simulink model "heating_system_model"  (R2022b)
settings: Solver=VariableStepAuto  StartTime=0.0  StopTime=500  RelTol=1e-3
model workspace (MAT data in the model file):
  h0 = [0 1 1 0]
  p0 = [0 1 1 0]
  x0 = [16.5 16.5 16.5 16.5]
settings Model: Creator=Cameron  LastModifiedBy=Cameron

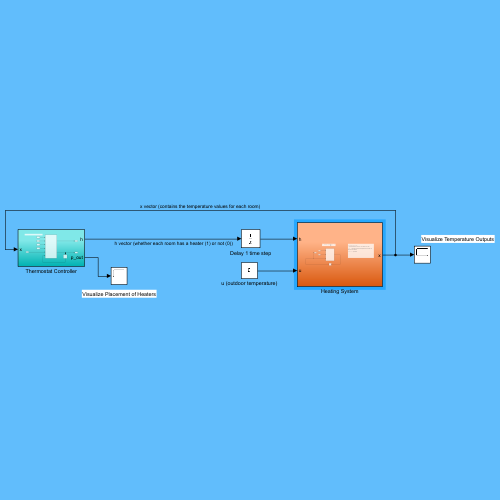
[thumbnail: Simulink's stored preview of the top-level diagram]
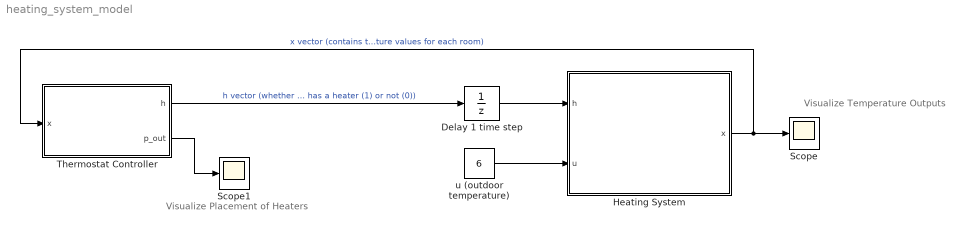
== system heating_system_model ==
  note: Visualize Placement of Heaters
  note: Visualize Temperature Outputs
  Delay 1 time step : UnitDelay  SampleTime=-1  HasFrameUpgradeWarning=on
  Heating System : Subsystem
  Scope : Scope
  Scope1 : Scope
  Thermostat Controller : Subsystem
  u (outdoor temperature) : Constant  Value=6
  wires:
  Thermostat Controller/1(h) -> Delay 1 time step/1  "h vector (whether each room has a heater (1) or not (0))"
  Heating System/1(x) -> Scope/1, Thermostat Controller/1(x)  "x vector (contains the temperature values for each room)"
  u (outdoor temperature)/1 -> Heating System/2(u)
  Delay 1 time step/1 -> Heating System/1(h)
  Thermostat Controller/2(p_out) -> Scope1/1

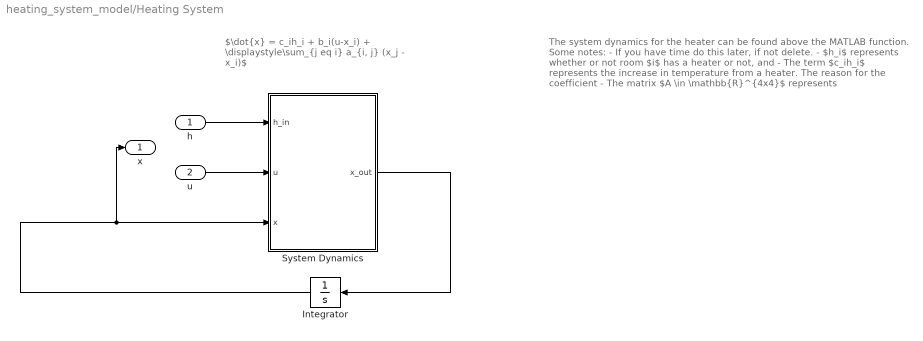
== system heating_system_model/Heating System ==
  note: The system dynamics for the heater can be found above the MATLAB function. Some notes:
      |
      | - If you have time do this later, if not delete.
      |
      | - $h_i$ represents whether or not room $i$ has a heater or not, and
      |
      | - The term $c_ih_i$ represents the increase in temperature from a heater. The reason for the coefficient
      |
      | - The matrix $A \in \mathbb{R}^{4x4}$ represents
  note: $\dot{x} = c_ih_i + b_i(u-x_i) + \displaystyle\sum_{j \neq i} a_{i, j} (x_j - x_i)$
  h : Inport  PortDimensions=4
  u : Inport  Port=2
  Integrator : Integrator  InitialCondition=x0
  System Dynamics : MATLAB Function  TreatAsAtomicUnit=on
  x : Outport  PortDimensions=4
  wires:
  h/1 -> System Dynamics/1(h_in)
  u/1 -> System Dynamics/2(u)
  Integrator/1 -> x/1, System Dynamics/3(x)
  System Dynamics/1(x_out) -> Integrator/1

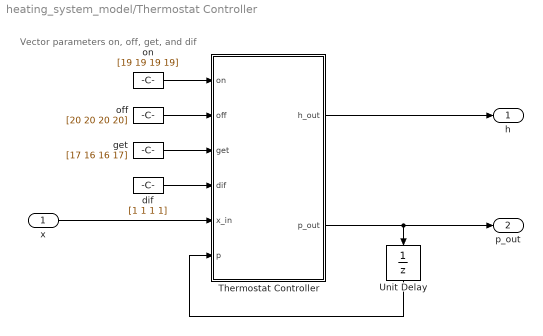
== system heating_system_model/Thermostat Controller ==
  note: Vector parameters on, off, get, and dif
  x : Inport  PortDimensions=4
  Thermostat Controller : MATLAB Function  TreatAsAtomicUnit=on
  Unit Delay : UnitDelay  InitialCondition=p0  SampleTime=-1  HasFrameUpgradeWarning=on
  dif : Constant  Value=[1 1 1 1]
  get : Constant  Value=[17 16 16 17]
  off : Constant  Value=[20 20 20 20]
  on : Constant  Value=[19 19 19 19]
  h : Outport  PortDimensions=4
  p_out : Outport  Port=2
  wires:
  x/1 -> Thermostat Controller/5(x_in)
  Thermostat Controller/1(h_out) -> h/1
  on/1 -> Thermostat Controller/1(on)
  get/1 -> Thermostat Controller/3(get)
  dif/1 -> Thermostat Controller/4(dif)
  off/1 -> Thermostat Controller/2(off)
  Unit Delay/1 -> Thermostat Controller/6(p)
  Thermostat Controller/2(p_out) -> p_out/1, Unit Delay/1

== matlab function heating_system_model/Thermostat Controller/Thermostat Controller ==
  data: on input; off input; get input; dif input; x_in input; h_out output; p input; p_out output
% This function moves the heaters according to the specification.
% It returns h, which is a required output for the heating system.
% It also returns p_out, which is the variable we need to figure out where
%     to move the heaters.
% The variable p represents simply if there is a heater in room i.
% h is an extension where the heater has to be on for the value to
%     be 1.

function [h_out,p_out] = fcn(on, off, get, dif, x_in, p)

% for a heater to be moved to room i, x_i <= get_i
% in other words, x_i - get_i <= 0
% in English, the room has to be cold enough to require the heater

% for a heater to be moved from j to i, x_j - x_i >= dif_i
% in other words, the difference between the two rooms must be big enough
%     for room j to give up its heater

% we assume that only one heater can be moved at a time
% if a heater can be moved to two different rooms or two heaters can be
%     moved to the same room, just pick an arbitrary one to move
% this was given in the specifications; we can decide however we want
% there is probably a better algorithmic way to do this, but I will keep it
%     simple for this project (e.g., take the argmin of x - g and choose
%     the best room to move and give up the heaters)
% move the heater from j to i
p_out = p'; % initialize to the original value
for i = 1:length(p)
    for j = 1:length(p)
        if (0 == p(i) && 1 == p(j)) % there's a heater in room j, not i
            if (x_in(i) <= get(i) && x_in(j) - x_in(i) >= dif(i))
                
                % we can move the heater from room j to room i
                % simply update the indices of p
                % select the first available heater to move
                p_out(i) = 1;
                p_out(j) = 0;

            end
        end
    end
end

% finally, compute the h value for each room
% a value of 1 means that (a) there is a heater in the room and (b) the
%     heater is turned on
% we will use p_out and the constants on and off to compute this
h_out = zeros(4, 1);
for i = 1:length(p_out)
    if (1 == p_out(i) && x_in(i) <= on(i))
        h_out(i) = 1;
    end
end

% to be sure we are following the specs, we will check the off variable too
% I don't think we actually need this, but if the temperature is greater
%     than the off constant, the heater is off.
for i = 1:length(p_out)
    if (x_in(i) >= off(i))
        h_out(i) = 0;
    end
end

disp(p);
disp(p_out);

== matlab function heating_system_model/Heating System/System Dynamics ==
  data: h_in input; x_out output; u input; x input
% This function defines the dynamics for the heating system
% The dynamics are defined in the specification

function x_out = fcn(h_in, u, x)
 
% step 1: define constants from specification
% This includes matrix A, and vectors b and c
% We will define these constants in this function because they are only
%    used for the system dynamics (e.g., in this subsystem)
% change these parameters for different simulations

% The matrix A represents the configuration of the 4 rooms
% E.g., how "close" each room is to every other
% This is a general way of describing the relationship between the rooms
A = [0 0.3 0.4 0.3; 0.3 0 0.5 0; 0.4 0.5 0 0.3; 0.3 0 0.3 0];

% The vector b defines the relationship between each room and outside
% we multiply b(u - x_i)
% therefore, this vector represents how "close" each room is to outside
% a higher b value means it's closer and will be changed more by
%     temperature outside
b = [0.3 0.2 0.5 0.4];

% The vector c defines the relative size of each room
% A larger c value for a room means the heater will increase the
%     temperature more
% we can think of this as the room being smaller, since there's less space
%     to heat
c = [9 7 11 7];

% step 2: compute the dynamics of the system
% there is an update for each element of the vector x
% again, see specification for this calculation
x_out = zeros(1, 4);
for i = 1:length(h_in)

    % calculate increase in temperature due to heater
    term1 = c(i) * h_in(i);

    % calculate decrease in room temperature from outdoor temperature
    term2 = b(i) * (u - x(i));

    % calculate change in temperature from other rooms
    term3 = 0;
    for j = 1:length(h_in)
        if (j ~= i)
            term3 = term3 + A(i, j) * (x(j) - x(i));
        end
    end

    % place sum into correct index of x_out
    % note that the calculation is for the CHANGE in temperature, not the
    %     overall new temperature
    scale_factor = 0.15;
    x_out(i) = scale_factor * (term1 + term2 + term3);
end
